simulink model "RegulationPDJointSpace"  (R2019a)
settings: Solver=VariableStepAuto  StartTime=0.0  StopTime=40  RelTol=1e-3
libraries: simulink x4, dspinverses x1
settings Model: Creator=amir  LastModifiedBy=amir
settings DataIOCC: ReturnWorkspaceOutputs=off

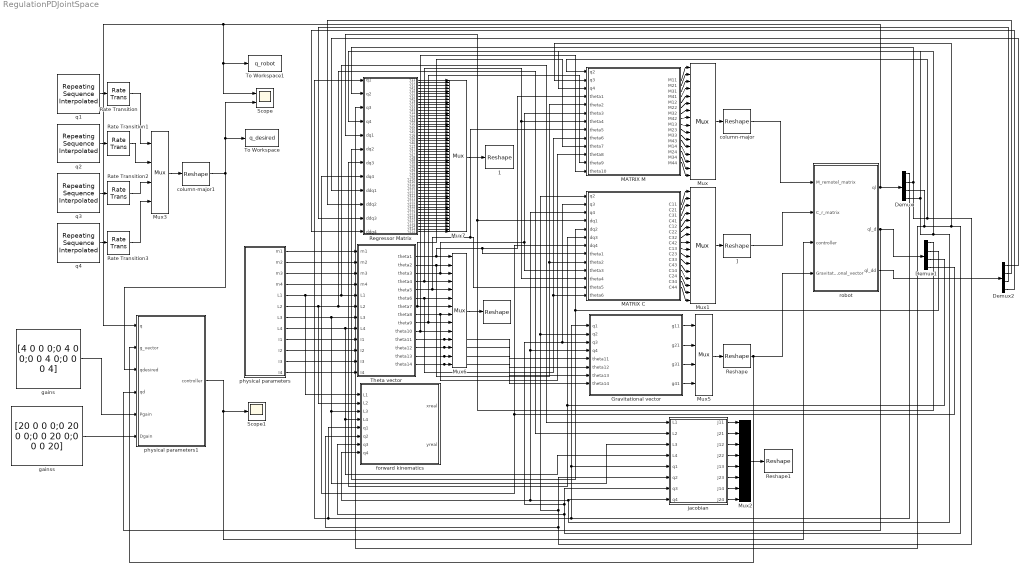
== system RegulationPDJointSpace ==
  " " : Reshape  OutputDimensionality=Customize  OutputDimensions=[14,1]
  " 1" : Reshape  OutputDimensionality=Customize  OutputDimensions=[4,14]
  " ] " : Reshape  OutputDimensionality=Customize  OutputDimensions=[4,4]
  Demux : Demux
  Demux1 : Demux
  Demux2 : Demux
  Gravitational vector : MATLAB Function  TreatAsAtomicUnit=on
  MATRIX C : MATLAB Function  TreatAsAtomicUnit=on
  MATRIX M : MATLAB Function  TreatAsAtomicUnit=on
  Mux : Mux  Inputs=16
  Mux1 : Mux  Inputs=16
  Mux2 : Mux  Inputs=8
  Mux3 : Mux
  Mux5 : Mux
  Mux6 : Mux  Inputs=14
  Mux7 : Mux  Inputs=56
  Rate Transition{,1..3} (4 alike) : RateTransition
  Regressor Matrix : MATLAB Function  TreatAsAtomicUnit=on
  Reshape : Reshape  OutputDimensionality=Customize  OutputDimensions=[4,1]
  Reshape1 : Reshape  OutputDimensionality=Customize  OutputDimensions=[2,4]
  Scope : Scope  NumInputPorts=2
  Scope1 : Scope
  Theta vector : MATLAB Function  TreatAsAtomicUnit=on
  To Workspace : ToWorkspace  VariableName=q_desired  SaveFormat=Timeseries  SampleTime=-1
  To Workspace1 : ToWorkspace  VariableName=q_robot  SaveFormat=Timeseries  SampleTime=-1
  column-major : Reshape  OutputDimensionality=Customize  OutputDimensions=[4,4]
  column-major1 : Reshape  OutputDimensionality=Customize  OutputDimensions=[4,1]
  forward kinematics : MATLAB Function  TreatAsAtomicUnit=on
  gains : Constant  Value=[4 0 0 0;0 4 0 0;0 0 4 0;0 0 0 4]
  "gainss " : Constant  Value=[20 0 0 0;0 20 0 0;0 0 20 0;0 0 0 20]
  jacobian : MATLAB Function  TreatAsAtomicUnit=on
  physical parameters : MATLAB Function  TreatAsAtomicUnit=on
  physical parameters1 : MATLAB Function  TreatAsAtomicUnit=on
  q{1..4} (4 alike) : simulink/Sources/Repeating Sequence Interpolated  OutValues=1.046*[1 1].'  TimeValues=[0 40].'  LookUpMeth=Interpolation-Use End Values  tsamp=0.01  OutMin=[]  OutMax=[]  OutDataTypeStr=float('double')  OutputDataTypeScalingMode=Specify via dialog  OutDataType=float('double')  OutScaling=2^-10
  robot : Subsystem
  wires:
  Mux/1 -> column-major/1
  MATRIX M/1(M11) -> Mux/1
  MATRIX M/2(M21) -> Mux/2
  MATRIX M/3(M31) -> Mux/3
  MATRIX M/4(M41) -> Mux/4
  MATRIX M/5(M12) -> Mux/5
  MATRIX M/6(M22) -> Mux/6
  MATRIX M/7(M32) -> Mux/7
  MATRIX M/8(M42) -> Mux/8
  MATRIX M/9(M13) -> Mux/9
  MATRIX M/10(M23) -> Mux/10
  MATRIX M/11(M33) -> Mux/11
  MATRIX M/12(M43) -> Mux/12
  MATRIX M/13(M14) -> Mux/13
  MATRIX M/14(M24) -> Mux/14
  MATRIX M/15(M34) -> Mux/15
  MATRIX M/16(M44) -> Mux/16
  MATRIX C/1(C11) -> Mux1/1
  MATRIX C/2(C21) -> Mux1/2
  MATRIX C/3(C31) -> Mux1/3
  MATRIX C/4(C41) -> Mux1/4
  MATRIX C/5(C12) -> Mux1/5
  MATRIX C/6(C22) -> Mux1/6
  MATRIX C/7(C32) -> Mux1/7
  MATRIX C/8(C42) -> Mux1/8
  MATRIX C/9(C13) -> Mux1/9
  MATRIX C/10(C23) -> Mux1/10
  MATRIX C/11(C33) -> Mux1/11
  MATRIX C/12(C43) -> Mux1/12
  MATRIX C/13(C14) -> Mux1/13
  MATRIX C/14(C24) -> Mux1/14
  MATRIX C/15(C34) -> Mux1/15
  MATRIX C/16(C44) -> Mux1/16
  Mux1/1 -> " ] "/1
  Gravitational vector/1(g11) -> Mux5/1
  Gravitational vector/2(g21) -> Mux5/2
  Gravitational vector/3(g31) -> Mux5/3
  Gravitational vector/4(g41) -> Mux5/4
  Mux5/1 -> Reshape/1
  Theta vector/1(theta1) -> MATRIX M/4(theta1), MATRIX C/8(theta1), Mux6/1
  Theta vector/2(theta2) -> MATRIX M/5(theta2), MATRIX C/9(theta2), Mux6/2
  Theta vector/3(theta3) -> MATRIX M/6(theta3), MATRIX C/10(theta3), Mux6/3
  Theta vector/4(theta4) -> MATRIX M/7(theta4), MATRIX C/11(theta4), Mux6/4
  Theta vector/5(theta5) -> MATRIX M/8(theta5), MATRIX C/12(theta5), Mux6/5
  Theta vector/6(theta6) -> MATRIX M/9(theta6), MATRIX C/13(theta6), Mux6/6
  Theta vector/7(theta7) -> MATRIX M/10(theta7), Mux6/7
  Theta vector/8(theta8) -> MATRIX M/11(theta8), Mux6/8
  Theta vector/9(theta9) -> MATRIX M/12(theta9), Mux6/9
  Theta vector/10(theta10) -> MATRIX M/13(theta10), Mux6/10
  Theta vector/11(theta11) -> Gravitational vector/5(theta11), Mux6/11
  Theta vector/12(theta12) -> Gravitational vector/6(theta12), Mux6/12
  Theta vector/13(theta13) -> Gravitational vector/7(theta13), Mux6/13
  Theta vector/14(theta14) -> Gravitational vector/8(theta14), Mux6/14
  Mux6/1 -> " "/1
  Regressor Matrix/1(Y11) -> Mux7/1
  Regressor Matrix/2(Y21) -> Mux7/2
  Regressor Matrix/3(Y31) -> Mux7/3
  Regressor Matrix/4(Y41) -> Mux7/4
  Regressor Matrix/5(Y12) -> Mux7/5
  Regressor Matrix/6(Y22) -> Mux7/6
  Regressor Matrix/7(Y32) -> Mux7/7
  Regressor Matrix/8(Y42) -> Mux7/8
  Regressor Matrix/9(Y13) -> Mux7/9
  Regressor Matrix/10(Y23) -> Mux7/10
  Regressor Matrix/11(Y33) -> Mux7/11
  Regressor Matrix/12(Y43) -> Mux7/12
  Regressor Matrix/13(Y14) -> Mux7/13
  Regressor Matrix/14(Y24) -> Mux7/14
  Regressor Matrix/15(Y34) -> Mux7/15
  Regressor Matrix/16(Y44) -> Mux7/16
  Regressor Matrix/17(Y15) -> Mux7/17
  Regressor Matrix/18(Y25) -> Mux7/18
  Regressor Matrix/19(Y35) -> Mux7/19
  Regressor Matrix/20(Y45) -> Mux7/20
  Regressor Matrix/21(Y16) -> Mux7/21
  Regressor Matrix/22(Y26) -> Mux7/22
  Regressor Matrix/23(Y36) -> Mux7/23
  Regressor Matrix/24(Y46) -> Mux7/24
  Regressor Matrix/25(Y17) -> Mux7/25
  Regressor Matrix/26(Y27) -> Mux7/26
  Regressor Matrix/27(Y37) -> Mux7/27
  Regressor Matrix/28(Y47) -> Mux7/28
  Regressor Matrix/29(Y18) -> Mux7/29
  Regressor Matrix/30(Y28) -> Mux7/30
  Regressor Matrix/31(Y38) -> Mux7/31
  Regressor Matrix/32(Y48) -> Mux7/32
  Regressor Matrix/33(Y19) -> Mux7/33
  Regressor Matrix/34(Y29) -> Mux7/34
  Regressor Matrix/35(Y39) -> Mux7/35
  Regressor Matrix/36(Y49) -> Mux7/36
  Regressor Matrix/37(Y110) -> Mux7/37
  Regressor Matrix/38(Y210) -> Mux7/38
  Regressor Matrix/39(Y310) -> Mux7/39
  Regressor Matrix/40(Y410) -> Mux7/40
  Regressor Matrix/41(Y111) -> Mux7/41
  Regressor Matrix/42(Y211) -> Mux7/42
  Regressor Matrix/43(Y311) -> Mux7/43
  Regressor Matrix/44(Y411) -> Mux7/44
  Regressor Matrix/45(Y112) -> Mux7/45
  Regressor Matrix/46(Y212) -> Mux7/46
  Regressor Matrix/47(Y312) -> Mux7/47
  Regressor Matrix/48(Y412) -> Mux7/48
  Regressor Matrix/49(Y113) -> Mux7/49
  Regressor Matrix/50(Y213) -> Mux7/50
  Regressor Matrix/51(Y313) -> Mux7/51
  Regressor Matrix/52(Y413) -> Mux7/52
  Regressor Matrix/53(Y114) -> Mux7/53
  Regressor Matrix/54(Y214) -> Mux7/54
  Regressor Matrix/55(Y314) -> Mux7/55
  Regressor Matrix/56(Y414) -> Mux7/56
  Mux7/1 -> " 1"/1
  column-major/1 -> robot/1(M_remotel_matrix)
  " ] "/1 -> robot/2(C_r_matrix)
  Reshape/1 -> physical parameters1/2(g_vector), robot/4(Gravitational_vector)
  robot/2(ql_d) -> physical parameters1/4(qd), Demux1/1
  robot/1(ql) -> To Workspace1/1, Scope/1, physical parameters1/1(q), Demux/1
  physical parameters/1(m1) -> Theta vector/1(m1)
  physical parameters/2(m2) -> Theta vector/2(m2)
  physical parameters/3(m3) -> Theta vector/3(m3)
  physical parameters/4(m4) -> Theta vector/4(m4)
  physical parameters/5(L1) -> forward kinematics/1(L1), Theta vector/5(L1), jacobian/1(L1)
  physical parameters/6(L2) -> forward kinematics/2(L2), Theta vector/6(L2), jacobian/2(L2)
  physical parameters/7(L3) -> jacobian/3(L3), forward kinematics/3(L3), Theta vector/7(L3)
  physical parameters/8(L4) -> jacobian/4(L4), forward kinematics/4(L4), Theta vector/8(L4)
  physical parameters/9(I1) -> Theta vector/9(I1)
  physical parameters/10(I2) -> Theta vector/10(I2)
  physical parameters/11(I3) -> Theta vector/11(I3)
  physical parameters/12(I4) -> Theta vector/12(I4)
  Demux/1 -> forward kinematics/5(q1), Regressor Matrix/1(q1), jacobian/5(q1), Gravitational vector/1(q1)
  Demux/2 -> MATRIX M/1(q2), MATRIX C/1(q2), Gravitational vector/2(q2), jacobian/6(q2), forward kinematics/6(q2), Regressor Matrix/2(q2)
  Demux/3 -> Regressor Matrix/3(q3), MATRIX M/2(q3), MATRIX C/2(q3), Gravitational vector/3(q3), jacobian/7(q3), forward kinematics/7(q3)
  Demux/4 -> MATRIX M/3(q4), MATRIX C/3(q4), Gravitational vector/4(q4), forward kinematics/8(q4), jacobian/8(q4), Regressor Matrix/4(q4)
  jacobian/1(J11) -> Mux2/1
  jacobian/2(J21) -> Mux2/2
  jacobian/3(J12) -> Mux2/3
  jacobian/4(J22) -> Mux2/4
  jacobian/5(J13) -> Mux2/5
  jacobian/6(J23) -> Mux2/6
  jacobian/7(J14) -> Mux2/7
  jacobian/8(J24) -> Mux2/8
  Mux2/1 -> Reshape1/1
  Demux1/1 -> Regressor Matrix/5(dq1), MATRIX C/4(dq1)
  Demux1/2 -> MATRIX C/5(dq2), Regressor Matrix/6(dq2)
  Demux1/3 -> MATRIX C/6(dq3), Regressor Matrix/7(dq3)
  Demux1/4 -> MATRIX C/7(dq4), Regressor Matrix/8(dq4)
  robot/3(ql_dd) -> Demux2/1
  Demux2/1 -> Regressor Matrix/9(ddq1)
  Demux2/2 -> Regressor Matrix/10(ddq2)
  Demux2/3 -> Regressor Matrix/11(ddq3)
  Demux2/4 -> Regressor Matrix/12(ddq4)
  q1/1 -> Rate Transition/1
  q2/1 -> Rate Transition1/1
  q4/1 -> Rate Transition3/1
  q3/1 -> Rate Transition2/1
  Rate Transition/1 -> Mux3/1
  Rate Transition1/1 -> Mux3/2
  Rate Transition2/1 -> Mux3/3
  Rate Transition3/1 -> Mux3/4
  Mux3/1 -> column-major1/1
  column-major1/1 -> To Workspace/1, Scope/2, physical parameters1/3(qdesired)
  physical parameters1/1(controller) -> Scope1/1, robot/3(controller)
  gains/1 -> physical parameters1/5(Pgain)
  "gainss "/1 -> physical parameters1/6(Dgain)

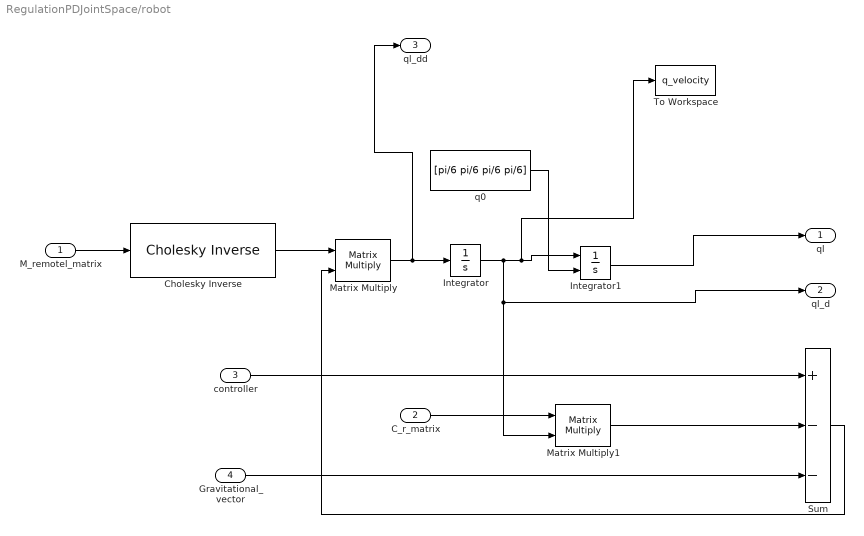
== system RegulationPDJointSpace/robot ==
  M_remotel_matrix : Inport
  C_r_matrix : Inport  Port=2
  controller : Inport  Port=3
  Gravitational_vector : Inport  Port=4
  Cholesky Inverse : dspinverses/Cholesky Inverse  errmode=Warning
      settings: SourceProductName=DSP System Toolbox  SourceProductBaseCode=DS
  Integrator : Integrator
  Integrator1 : Integrator  InitialConditionSource=external
  Matrix Multiply : Product  Multiplication=Matrix(*)
  Matrix Multiply1 : Product  Multiplication=Matrix(*)
  Sum : Sum  Inputs=+--
  To Workspace : ToWorkspace  VariableName=q_velocity  SaveFormat=Timeseries  SampleTime=-1
  q0 : Constant  Value=[pi/6 pi/6 pi/6 pi/6]
  ql : Outport
  ql_d : Outport  Port=2
  ql_dd : Outport  Port=3
  wires:
  Matrix Multiply1/1 -> Sum/2
  M_remotel_matrix/1 -> Cholesky Inverse/1
  Integrator/1 -> ql_d/1, Matrix Multiply1/2, To Workspace/1, Integrator1/1
  q0/1 -> Integrator1/2
  Cholesky Inverse/1 -> Matrix Multiply/1
  Matrix Multiply/1 -> ql_dd/1, Integrator/1
  controller/1 -> Sum/1
  Integrator1/1 -> ql/1
  Sum/1 -> Matrix Multiply/2
  C_r_matrix/1 -> Matrix Multiply1/1
  Gravitational_vector/1 -> Sum/3

== matlab function RegulationPDJointSpace/MATRIX C ==
  data: q2 input; q3 input; C11 output; q4 input; dq1 input; dq2 input; dq3 input; C21 output; C31 output; C41 output; C12 output; C22 output; dq4 input; C32 output; C42 output; C13 output; C23 output; C33 output; C43 output; C14 output; C24 output; C34 output; C44 output; theta1 input; theta2 input; theta3 input; theta4 input; theta5 input; theta6 input
function [C11, C21, C31, C41, ...
    C12, C22, C32, C42, ...
    C13, C23, C33, C43, ....
    C14, C24, C34, C44] = fcn(q2,q3,q4,dq1,dq2,dq3,dq4, ...
    theta1,theta2,theta3,theta4,theta5,theta6)
s2 = sin(q2);
s23 = sin(q2+q3);
s234 = sin(q2+q3+q4);
s3 = sin(q3);
s34 = sin(q3+q4);
s4 = sin(q4);
%%%
dq12 = dq1+dq2;
dq123 = dq1+dq2+dq3;
dq1234 = dq1+dq2+dq3+dq4;
dq23 = dq2+dq3;
dq234 = dq2+dq3+dq4;
dq34 = dq3+dq4;
dq1_2 = dq1-dq2;
%%%
C11 = -dq2*s2*theta1-dq23*s23*theta2-dq234*s234*theta3- ...
    dq3*s3*theta4-dq34*s34*theta5-dq4*s4*theta6;
C12 = -dq12*s2*theta1-dq123*s23*theta2-dq1234*s234*theta3- ...
    dq3*s3*theta4-dq34*s34*theta5-dq4*s4*theta6;
C13 = dq123*s23*theta2-dq1234*s234*theta3-dq123*s3*theta4- ...
    dq1234*s34*theta5-dq4*s4*theta6;
C14 = -dq1234*s234*theta3-dq1234*s34*theta5-dq1234*s4*theta6;
C21 = dq1*s2*theta1+dq1*s23*theta2+dq1*s234*theta3-dq3*s3*theta4- ...
    dq34*s34*theta5-dq4*s4*theta6;
C22 = -dq3*s3*theta4-dq34*s34*theta5-dq4*s4*theta6;
C23 = -dq123*s3*theta4-dq1234*s34*theta5-dq4*s4*theta6;
C24 = -dq1234*s34*theta5-dq1234*s4*theta6;
C31 = -dq1*s23*theta2-dq1*s234*theta3-dq1_2*s3*theta4- ...
    dq1_2*s34*theta5-dq4*s4*theta6;
C32 = dq12*s3*theta4+dq12*s34*theta5-dq4*s4*theta6;
C33 = -dq4*s4*theta6;
C34 = -dq1234*s4*theta6;
C41 = dq1*s234*theta3+dq12*s34*theta5+dq123*s4*theta6;
C42 = dq12*s34*theta5+dq123*s4*theta5;
C43 = dq123*s4*theta6;
C44 = 0;

== matlab function RegulationPDJointSpace/MATRIX M ==
  data: q2 input; q3 input; q4 input; theta1 input; theta2 input; theta3 input; theta4 input; theta5 input; theta6 input; theta7 input; theta8 input; M11 output; M21 output; M31 output; M41 output; theta9 input; theta10 input; M12 output; M22 output; M32 output; M42 output; M13 output; M23 output; M33 output; M43 output; M14 output; M24 output; M34 output; M44 output
function [M11, M21, M31, M41, ...
    M12, M22, M32, M42, ...
    M13, M23, M33, M43, ...
    M14, M24, M34, M44] = fcn(q2,q3,q4,theta1,theta2,theta3,theta4,theta5,theta6,theta7,theta8,theta9,theta10)

%%%
c2 = cos(q2);
c23 = cos(q2+q3);
c234 = cos(q2+q3+q4);
c3 = cos(q3);
c34 = cos(q3+q4);
c4 = cos(q4);
M11 = 2*c2*theta1+2*c23*theta2+2*c234*theta3+2*c3*theta4+ ... 
    2*c34*theta5+2*c4*theta6+theta7;
M21 = c2*theta1+c23*theta2+c234*theta3+2*c3*theta4+...
    2*c34*theta5+2*c4*theta6+theta8;
M31 = c23*theta2+c234*theta3+c3*theta4+c34*theta5+2*c4*theta6+theta9;
M41 = c234*theta3+c34*theta5+c4*theta6+theta10;
M12 = M21;
M22 = 2*c3*theta4+2*c34*theta5+2*c4*theta6+theta8;
M32 = c3*theta4+c34*theta5+2*c4*theta6+theta9;
M42 = c34*theta5+c4*theta6+theta10;
M13 = M31;
M23 = M32;
M33 = 2*c4*theta6+theta9;
M43 = c4*theta6+theta10;
M14 = M41;
M24 = M42;
M34 = M43;
M44 = theta10;

== matlab function RegulationPDJointSpace/forward kinematics ==
  data: L1 input; L2 input; L3 input; L4 input; q1 input; xreal output; q2 input; yreal output; q3 input; q4 input
function [xreal, yreal] = fcn(L1,L2,L3,L4,q1,q2,q3,q4)
q12=q1+q2;
q123=q1+q2+q3;
q1234=q1+q2+q3+q4;
%%%
xreal = L1*cos(q1)+L2*cos(q12)+L3*cos(q123)+L4*cos(q1234);
yreal = L1*sin(q1)+L2*sin(q12)+L3*sin(q123)+L4*sin(q1234);

== matlab function RegulationPDJointSpace/physical parameters ==
  data: m1 output; m2 output; m3 output; m4 output; L1 output; L2 output; L3 output; L4 output; I1 output; I2 output; I3 output; I4 output
function [m1, m2, m3, m4, L1, L2, L3, L4, I1, I2, I3, I4] = fcn()
m1 = 1;
m2 = 1;
m3 = 1;
m4 = 1;
%%%
L1 = 1;
L2 = 1;
L3 = 1;
L4 = 1;
%%%
I1 = 0.1;
I2 = 0.1;
I3 = 0.1;
I4 = 0.1;

== matlab function RegulationPDJointSpace/jacobian ==
  data: L1 input; L2 input; L3 input; L4 input; q1 input; J11 output; q2 input; J21 output; J12 output; J22 output; q3 input; q4 input; J13 output; J23 output; J14 output; J24 output
function [J11, J21, J12, J22, J13, J23, J14, J24] = fcn(L1,L2,L3,L4,q1,q2,q3,q4)
%%%
q12=q1+q2;
q123=q1+q2+q3;
q1234=q1+q2+q3+q4;
%%%
J11=-L1*sin(q1)-L2*sin(q12)-L3*sin(q123)-L4*sin(q1234);
J21=L1*cos(q1)+L2*cos(q12)+L3*cos(q123)+L4*cos(q1234);
%%%
J12=-L2*sin(q12)-L3*sin(q123)-L4*sin(q1234);
J22=L2*cos(q12)+L3*cos(q123)+L4*cos(q1234);
%%%
J13=-L3*sin(q123)-L4*sin(q1234);
J23=L3*cos(q123)+L4*cos(q1234);
%%%
J14=-L4*sin(q1234);
J24=L4*cos(q1234);

== matlab function RegulationPDJointSpace/Theta vector ==
  data: m1 input; m2 input; m3 input; m4 input; theta1 output; theta2 output; L1 input; L2 input; L3 input; L4 input; theta3 output; theta4 output; I1 input; I2 input; I3 input; I4 input; theta5 output; theta6 output; theta7 output; theta8 output; theta9 output; theta10 output; theta11 output; theta12 output; theta13 output; theta14 output
function [theta1, theta2, theta3, theta4, theta5, theta6, theta7, theta8, ...
    theta9, theta10, theta11, theta12, theta13, theta14] = ...
    fcn(m1,m2,m3,m4,L1,L2,L3,L4,I1,I2,I3,I4)
Lc1 = L1/2;
Lc2 = L2/2;
Lc3 = L3/2;
Lc4 = L4/2;
%%%
I1234 = I1+I2+I3+I4;
I234 = I2+I3+I4;
I34 = I3+I4;
%%%
L12 = L1+L2;
L123 = L1+L2+L3;
L1234 = L1+L2+L3+L4;
L23 = L2+L3;
L234=L2+L3+L4;
L34=L3+L4;
%%%
m234=m2+m3+m4;
m34=m3+m4;
%%%
theta1 = m2*L1*Lc2+m3*L1*L2+m4*L1*L2;
theta2 = m4*L1*L3+m3*L1*Lc3;
theta3 = m4*L1*Lc4;
theta4 = m3*L2*Lc3+m4*L2*L3;
theta5 = m4*L2*Lc4;
theta6 = m4*L3*Lc4;
theta7 = (m1*Lc1^2)+(m2*L12^2)+(m3*L123^2)+(m4*L1234^2)+I1234;
theta8 = (m2*Lc2^2)+(m3*L23^2)+(m4*L234^2)+I234;
theta9 = (m3*Lc3^2)+(m4*L34^2)+I34;
theta10 = (m4*Lc4^2)+I4;
theta11 = m1*Lc1+m234*L1;
theta12 = m2*Lc2+m34*L2;
theta13 = m3*Lc3+m4*L3;
theta14 = m4*Lc4;

== matlab function RegulationPDJointSpace/Gravitational vector ==
  data: q1 input; q2 input; q3 input; g11 output; q4 input; theta11 input; theta12 input; g21 output; g31 output; g41 output; theta13 input; theta14 input
function [g11,g21,g31,g41] = fcn(q1,q2,q3,q4,theta11,theta12,theta13,theta14)
%%%
g=9.81;
%%%
c1234 = cos(q1+q2+q3+q4);
c123 = cos(q1+q2+q3);
c12 = cos(q1+q2);
c1 = cos(q1);
%%%
g11 = g*c1*theta11+g*c12*theta12+g*c123*theta13+g*c1234*theta14;
g21 = g*c12*theta12+g*c123*theta13+g*c1234*theta14;
g31 = g*c123*theta13+g*c1234*theta14;
g41 = g*c1234*theta14;

== matlab function RegulationPDJointSpace/Regressor Matrix ==
  data: q1 input; q2 input; q3 input; q4 input; dq1 input; dq2 input; dq3 input; dq4 input; ddq1 input; ddq2 input; ddq3 input; ddq4 input; Y11 output; Y21 output; Y31 output; Y41 output; Y12 output; Y22 output; Y32 output; Y42 output; Y13 output; Y23 output; Y33 output; Y43 output; Y14 output; Y24 output; Y34 output; Y44 output; Y15 output; Y25 output; Y35 output; Y45 output; Y16 output; Y26 output; Y36 output; Y46 output; Y17 output; Y27 output; Y37 output; Y47 output; Y18 output; Y28 output; Y38 output; Y48 output; Y19 output; Y29 output; Y39 output; Y49 output; Y110 output; Y210 output; Y310 output; Y410 output; Y111 output; Y211 output; Y311 output; Y411 output; Y112 output; Y212 output; Y312 output; Y412 output; Y113 output; Y213 output; Y313 output; Y413 output; Y114 output; Y214 output; Y314 output; Y414 output
function [Y11, Y21, Y31, Y41, ...
    Y12, Y22, Y32, Y42, ...
    Y13, Y23, Y33, Y43, ...
    Y14, Y24, Y34, Y44, ...
    Y15, Y25, Y35, Y45, ...
    Y16, Y26, Y36, Y46, ...
    Y17, Y27, Y37, Y47, ...
    Y18, Y28, Y38, Y48, ...
    Y19, Y29, Y39, Y49, ...
    Y110, Y210, Y310, Y410, ...
    Y111, Y211, Y311, Y411, ...
    Y112, Y212, Y312, Y412, ...
    Y113, Y213, Y313, Y413, ...
    Y114, Y214, Y314, Y414] = fcn(q1,q2,q3,q4,dq1,dq2,dq3,dq4, ...
    ddq1,ddq2,ddq3,ddq4)

%%%
g=9.81;
%%%
c1 = cos(q1);
c2 = cos(q2);
c12 = cos(q1+q2);
c123 = cos(q1+q2+q3);
c1234 = cos(q1+q2+q3+q4);
c23 = cos(q2+q3);
c234 = cos(q2+q3+q4);
c3 = cos(q3);
c34 = cos(q3+q4);
c4 = cos(q4);
%%%
s2 = sin(q2);
s23 = sin(q2+q3);
s234 = sin(q2+q3+q4);
s3 = sin(q3);
s34 = sin(q3+q4);
s4 = sin(q4);
%%%
ddq1234 = ddq1+ddq2+ddq3+ddq4;
ddq123 = ddq1+ddq2+ddq3;
ddq12 = ddq1+ddq2;
ddq23 = ddq2+ddq3;
ddq34 = ddq3+ddq4;
ddq234 = ddq2+ddq3+ddq4;
dq123_2 = (dq1^2)+(dq2^2)+(dq3^2);
dq234_2 = (dq2^2)+(dq3^2)+(dq4^2);
dq34_2 = (dq3^2)+(dq4^2);
dq12_2 = (dq1^2)+(dq2^2);
dq1_dq234=dq1*(dq2+dq3+dq4);
dq1_dq34=dq1*(dq3+dq4);
dq1_dq23=dq1*(dq2+dq3);
dq2_dq34=dq2*(dq3+dq4);
dq3_dq12=dq3*(dq1+dq2);
dq4_dq123=dq4*(dq1+dq2+dq3);
%%%
Y11 =(2*ddq1+ddq2)*c2-(2*dq1*dq2+dq2^2)*s2 ;
Y12 = (2*ddq1+ddq23)*c23+(dq3^2-2*dq1*dq2-dq2^2)*s23;
Y13 = (2*ddq1+ddq234)*c234-(dq234_2+2*dq1_dq234+2*dq2_dq34+2*dq3*dq4)*s234;
Y14 = (2*ddq12+ddq3)*c3+(2*dq1*dq3+2*dq2*dq3+dq3^2)*s3;
Y15 = (2*ddq12+ddq34)*c34-(dq34_2+2*dq1_dq34+2*dq2_dq34+2*dq3*dq4)*s34;
Y16 = (2*ddq123+ddq4)*c4-(2*dq4_dq123+dq4^2)*s4;
Y17 = ddq1;
Y18 = ddq2;
Y19 = ddq3;
Y110 = ddq4;
Y111 = g*c1;
Y112 = g*c12;
Y113 = g*c123;
Y114 = g*c1234;
%%%
Y21 = (ddq1)*c2+(dq1^2)*s2;
Y22 = (ddq1)*c23+(dq1^2)*s23;
Y23 = (ddq1)*c234+(dq1^2)*s234;
Y24 = (2*ddq12+ddq3)*c3-(2*dq3_dq12+dq3^2)*s3;
Y25 = (2*ddq12+ddq34)*c34-(dq34_2+2*dq1_dq34+2*dq2_dq34+2*dq3*dq4)*s34;
Y26 = (2*ddq123+ddq4)*c4-(2*dq4_dq123+dq4^2)*s4;
Y27 = 0;
Y28 = ddq12;
Y29 = ddq3;
Y210 = ddq4;
Y211 = 0;
Y212 = g*c12;
Y213 = g*c123;
Y214 = g*c1234;
%%%
Y31 = 0;
Y32 = (ddq1)*c23-(dq1^2)*s23;
Y33 = (ddq1)*c234-(dq1^2)*s234;
Y34 = (ddq12)*c3+(2*dq1*dq2-dq1^2+dq2^2)*s3;
Y35 = (ddq12)*c34+(2*dq1*dq2-dq1^2+dq2^2)*s34;
Y36 = (2*ddq123+ddq4)*c4-(2*dq4_dq123+dq4^2)*s4;
Y37 = 0;
Y38 = 0;
Y39 = ddq123;
Y310 = ddq4;
Y311 = 0;
Y312 = 0;
Y313 = g*c123;
Y314 = g*c1234;
%%%
Y41 = 0;
Y42 = 0;
Y43 = (ddq1)*c234+(dq1^2)*s234;
Y44 = 0;
Y45 = (ddq12)*c34+(dq12_2+2*dq1*dq2)*s34;
Y46 = (ddq123)*c4+(dq123_2+2*dq1_dq23+2*dq2*dq3)*s4;
Y47 = 0;
Y48 = 0;
Y49 = 0;
Y410 = ddq1234;
Y411 = 0;
Y412 = 0;
Y413 = 0;
Y414 = g*c1234;

== matlab function RegulationPDJointSpace/physical parameters1 ==
  data: controller output; q input; g_vector input; qdesired input; qd input; Pgain input; Dgain input
function controller  = fcn(q,g_vector,qdesired,qd,Pgain,Dgain)
controller=g_vector+Pgain*(qdesired-q)-Dgain*qd;
